simulink model "testair"  (R2016b)
settings: Solver=VariableStepAuto  StartTime=0.0  StopTime=10.0  RelTol=1e-3
libraries: fl_lib x6, nesl_utility x6
(part 2 of 2)

== system testair/Subsystem1 ==
